simulink model "ADMIRE"  (R2021b)
settings: Solver=ode4  StartTime=0.0  StopTime=100  FixedStep=1e-2  RelTol=1e-3
undefined symbols (not defined in the file or in its folder): admireDB, Earth, WGS84
libraries: simulink_extras x112, simulink x27, aerolibutil x4, dspsigops x4, aerolibfltsims x3, sharedtransform x2, aerolibtransform2 x2, aerolibatmos2 x1, matrix_library x1, sharedutil x1, aerolibanimutils x1, vrlib x1
(part 5 of 15)

== system ADMIRE/Aircraft/Aerodynamics/NormalForceCoefficient/MachRegion3/Cncai ==
  in_bus : Inport
  Bus Selector : BusSelector  OutputSignals=AeroIn_Bus.angleOfAttack_deg,AeroIn_Bus.cai
  CNCAI_CAI_ALFA : Lookup_n-D  BreakpointsForDimension1=admireDB.aerodata_sym.CNCAI.breakpoints.ALFA  BreakpointsForDimension2=admireDB.aerodata_sym.CNCAI.breakpoints.CAI  BreakpointsForDimension3=[5, 7]  Table=admireDB.aerodata_sym.CNCAI.newTable  ExtrapMethod=Clip  InternalRulePriority=Speed  RndMeth=Simplest  InputSameDT=on
      settings: InputPortMap=u0,u1
  Cncai : Outport
  wires:
  CNCAI_CAI_ALFA/1 -> Cncai/1
  in_bus/1 -> Bus Selector/1  "in_bus"
  Bus Selector/2 -> CNCAI_CAI_ALFA/2  "<cai>"
  Bus Selector/1 -> CNCAI_CAI_ALFA/1  "<angleOfAttack_deg>"

== system ADMIRE/Aircraft/Aerodynamics/NormalForceCoefficient/MachRegion3/Cndedn ==
  Constant : Constant  Value=0
  Cndedn : Outport
  wires:
  Constant/1 -> Cndedn/1

== system ADMIRE/Aircraft/Aerodynamics/NormalForceCoefficient/MachRegion3/Cndei ==
  in_bus : Inport
  Bus Selector : BusSelector  OutputSignals=AeroIn_Bus.angleOfAttack_deg,AeroIn_Bus.dEI,AeroIn_Bus.mach_nd,eieff,AeroIn_Bus.qacorr
  CNEDEI_QA_M : Lookup_n-D  BreakpointsForDimension1=admireDB.aerodata_sym.CNEDEI.breakpoints.M  BreakpointsForDimension2=admireDB.aerodata_sym.CNEDEI.breakpoints.QA  BreakpointsForDimension3=[5, 7]  Table=admireDB.aerodata_sym.CNEDEI.newTable  ExtrapMethod=Clip  InternalRulePriority=Speed  RndMeth=Simplest  InputSameDT=on
      settings: InputPortMap=u0,u1
  Product : Product
  Subsystem : Subsystem
  Cndei : Outport
  wires:
  Product/1 -> Cndei/1
  Subsystem/1(Out1) -> Product/1
  Bus Selector/1 -> Subsystem/1(<angleOfAttack_deg>)  "<angleOfAttack_deg>"
  Bus Selector/2 -> Subsystem/2(<dEI>)  "<dEI>"
  Bus Selector/4 -> Subsystem/4(<eieff>)  "<eieff>"
  in_bus/1 -> Bus Selector/1  "in_bus"
  Bus Selector/5 -> CNEDEI_QA_M/2  "<qacorr>"
  Bus Selector/3 -> Subsystem/3(<mach_nd>), CNEDEI_QA_M/1  "<mach_nd>"
  CNEDEI_QA_M/1 -> Product/2

== system ADMIRE/Aircraft/Aerodynamics/NormalForceCoefficient/MachRegion3/Cndey ==
  in_bus : Inport
  Bus Selector : BusSelector  OutputSignals=AeroIn_Bus.angleOfAttack_deg,AeroIn_Bus.dEY,AeroIn_Bus.mach_nd,eieff,AeroIn_Bus.qacorr
  CNEDEY_QA_M : Lookup_n-D  BreakpointsForDimension1=admireDB.aerodata_sym.CNEDEY.breakpoints.M  BreakpointsForDimension2=admireDB.aerodata_sym.CNEDEY.breakpoints.QA  BreakpointsForDimension3=[5, 7]  Table=admireDB.aerodata_sym.CNEDEY.newTable  ExtrapMethod=Clip  InternalRulePriority=Speed  RndMeth=Simplest  InputSameDT=on
      settings: InputPortMap=u0,u1
  Product : Product
  Subsystem : Subsystem
  Cndey : Outport
  wires:
  CNEDEY_QA_M/1 -> Product/2
  Bus Selector/3 -> Subsystem/3(<mach_nd>), CNEDEY_QA_M/1  "<mach_nd>"
  Bus Selector/5 -> CNEDEY_QA_M/2  "<qacorr>"
  in_bus/1 -> Bus Selector/1  "in_bus"
  Bus Selector/4 -> Subsystem/4(<eieff>)  "<eieff>"
  Bus Selector/2 -> Subsystem/2(<dEI>)  "<dEY>"
  Bus Selector/1 -> Subsystem/1(<angleOfAttack_deg>)  "<angleOfAttack_deg>"
  Subsystem/1(Out1) -> Product/1
  Product/1 -> Cndey/1

== system ADMIRE/Aircraft/Aerodynamics/NormalForceCoefficient/MachRegion3/Cndle ==
  in_bus : Inport
  Bus Selector : BusSelector  OutputSignals=AeroIn_Bus.angleOfAttack_deg,AeroIn_Bus.mach_nd,AeroIn_Bus.lef_deg
  CNMDLEA_ALFA_DLE_M : Lookup_n-D  NumberOfTableDimensions=3  BreakpointsForDimension1=admireDB.aerodata_sym.CNMDLEA.breakpoints.ALFA  BreakpointsForDimension2=admireDB.aerodata_sym.CNMDLEA.breakpoints.DLE  BreakpointsForDimension3=admireDB.aerodata_sym.CNMDLEA.breakpoints.M  Table=admireDB.aerodata_sym.CNMDLEA.newTable  ExtrapMethod=Clip  InternalRulePriority=Speed  RndMeth=Simplest  InputSameDT=on
      settings: InputPortMap=u0,u1,u2
  Cndle : Outport
  wires:
  CNMDLEA_ALFA_DLE_M/1 -> Cndle/1
  Bus Selector/3 -> CNMDLEA_ALFA_DLE_M/3  "<lef_deg>"
  Bus Selector/2 -> CNMDLEA_ALFA_DLE_M/2  "<mach_nd>"
  Bus Selector/1 -> CNMDLEA_ALFA_DLE_M/1  "<angleOfAttack_deg>"
  in_bus/1 -> Bus Selector/1  "in_bus"

== system ADMIRE/Aircraft/Aerodynamics/NormalForceCoefficient/MachRegion3/Cndn ==
  in_bus : Inport
  Bus Selector : BusSelector  OutputSignals=AeroIn_Bus.dN,AeroIn_Bus.angleOfAttack_deg,AeroIn_Bus.mach_nd,AeroIn_Bus.qacorr
  CNDNH_M_DN_ALFA : Lookup_n-D  NumberOfTableDimensions=3  BreakpointsForDimension1=admireDB.aerodata_sym.CNDNH.breakpoints.M  BreakpointsForDimension2=admireDB.aerodata_sym.CNDNH.breakpoints.DN  BreakpointsForDimension3=admireDB.aerodata_sym.CNDNH.breakpoints.ALFA  Table=admireDB.aerodata_sym.CNDNH.newTable  ExtrapMethod=Clip  InternalRulePriority=Speed  RndMeth=Simplest  InputSameDT=on
      settings: InputPortMap=u0,u1,u2
  CNEDN_QA_M : Lookup_n-D  BreakpointsForDimension1=admireDB.aerodata_sym.CNEDN.breakpoints.M  BreakpointsForDimension2=admireDB.aerodata_sym.CNEDN.breakpoints.QA  BreakpointsForDimension3=[5, 7]  Table=admireDB.aerodata_sym.CNEDN.newTable  ExtrapMethod=Clip  InternalRulePriority=Speed  RndMeth=Simplest  InputSameDT=on
      settings: InputPortMap=u0,u1
  Product : Product
  Cndn : Outport
  wires:
  in_bus/1 -> Bus Selector/1  "in_bus"
  Bus Selector/1 -> CNDNH_M_DN_ALFA/2  "<dN>"
  Bus Selector/2 -> CNDNH_M_DN_ALFA/3  "<angleOfAttack_deg>"
  Bus Selector/4 -> CNEDN_QA_M/2  "<qacorr>"
  Bus Selector/3 -> CNDNH_M_DN_ALFA/1, CNEDN_QA_M/1  "<mach_nd>"
  CNEDN_QA_M/1 -> Product/2
  CNDNH_M_DN_ALFA/1 -> Product/1
  Product/1 -> Cndn/1

== system ADMIRE/Aircraft/Aerodynamics/NormalForceCoefficient/MachRegion3/Cnhigh ==
  Constant : Constant  Value=0
  Cnhigh : Outport
  wires:
  Constant/1 -> Cnhigh/1

== system ADMIRE/Aircraft/Aerodynamics/NormalForceCoefficient/MachRegion3/Cnlg ==
  in_bus : Inport
  Abs : Abs
  Bus Selector : BusSelector  OutputSignals=AeroIn_Bus.angleOfAttack_deg,AeroIn_Bus.angleOfSideslip_deg,AeroIn_Bus.lg_bool
  CNLST_BETA_ALFA : Lookup_n-D  BreakpointsForDimension1=admireDB.aerodata_sym.CNLST.breakpoints.ALFA  BreakpointsForDimension2=admireDB.aerodata_sym.CNLST.breakpoints.BETA  BreakpointsForDimension3=[5, 7]  Table=admireDB.aerodata_sym.CNLST.newTable  ExtrapMethod=Clip  InternalRulePriority=Speed  RndMeth=Simplest  InputSameDT=on
      settings: InputPortMap=u0,u1
  Product : Product
  Cnlg : Outport
  wires:
  Product/1 -> Cnlg/1
  in_bus/1 -> Bus Selector/1  "in_bus"
  Bus Selector/2 -> Abs/1  "<angleOfSideslip_deg>"
  Bus Selector/1 -> CNLST_BETA_ALFA/1  "<angleOfAttack_deg>"
  Abs/1 -> CNLST_BETA_ALFA/2
  CNLST_BETA_ALFA/1 -> Product/1
  Bus Selector/3 -> Product/2  "<lg_bool>"

== system ADMIRE/Aircraft/Aerodynamics/NormalForceCoefficient/MachRegion3/Cnnz ==
  in_bus : Inport
  Bus Selector : BusSelector  OutputSignals=AeroIn_Bus.nz_g,AeroIn_Bus.mach_nd,AeroIn_Bus.qacorr
  CNENZ_QA_M : Lookup_n-D  BreakpointsForDimension1=admireDB.aerodata_sym.CNENZ.breakpoints.M  BreakpointsForDimension2=admireDB.aerodata_sym.CNENZ.breakpoints.QA  BreakpointsForDimension3=[5, 7]  Table=admireDB.aerodata_sym.CNENZ.newTable  ExtrapMethod=Clip  InternalRulePriority=Speed  RndMeth=Simplest  InputSameDT=on
      settings: InputPortMap=u0,u1
  Constant : Constant
  Product : Product
  Sum : Sum  Inputs=-+|
  Cnnz : Outport
  wires:
  Bus Selector/2 -> CNENZ_QA_M/1  "<mach_nd>"
  Bus Selector/3 -> CNENZ_QA_M/2  "<qacorr>"
  Bus Selector/1 -> Sum/2  "<nz_g>"
  in_bus/1 -> Bus Selector/1  "in_bus"
  Product/1 -> Cnnz/1
  Constant/1 -> Sum/1
  Sum/1 -> Product/1
  CNENZ_QA_M/1 -> Product/2

== system ADMIRE/Aircraft/Aerodynamics/NormalForceCoefficient/MachRegion3/Cnq ==
  in_bus : Inport
  Bus Selector : BusSelector  OutputSignals=AeroIn_Bus.angleOfAttack_deg,AeroIn_Bus.qc,AeroIn_Bus.mach_nd,AeroIn_Bus.qacorr
  CNEQ_QA_M : Lookup_n-D  BreakpointsForDimension1=admireDB.aerodata_sym.CNEQ.breakpoints.M  BreakpointsForDimension2=admireDB.aerodata_sym.CNEQ.breakpoints.QA  BreakpointsForDimension3=[5, 7]  Table=admireDB.aerodata_sym.CNEQ.newTable  ExtrapMethod=Clip  InternalRulePriority=Speed  RndMeth=Simplest  InputSameDT=on
      settings: InputPortMap=u0,u1
  CNQAM_ALFA_M : Lookup_n-D  BreakpointsForDimension1=admireDB.aerodata_sym.CNQAM.breakpoints.M  BreakpointsForDimension2=admireDB.aerodata_sym.CNQAM.breakpoints.ALFA  BreakpointsForDimension3=[5, 7]  Table=admireDB.aerodata_sym.CNQAM.newTable  ExtrapMethod=Clip  InternalRulePriority=Speed  RndMeth=Simplest  InputSameDT=on
      settings: InputPortMap=u0,u1
  Product : Product  Inputs=3
  Cnq : Outport
  wires:
  CNQAM_ALFA_M/1 -> Product/1
  Product/1 -> Cnq/1
  in_bus/1 -> Bus Selector/1  "in_bus"
  Bus Selector/1 -> CNQAM_ALFA_M/2  "<angleOfAttack_deg>"
  Bus Selector/4 -> CNEQ_QA_M/2  "<qacorr>"
  Bus Selector/3 -> CNEQ_QA_M/1, CNQAM_ALFA_M/1  "<mach_nd>"
  CNEQ_QA_M/1 -> Product/3
  Bus Selector/2 -> Product/2  "<qc>"

== system ADMIRE/Aircraft/Aerodynamics/NormalForceCoefficient/MachRegion3/Cnqd ==
  in_bus : Inport
  Bus Selector : BusSelector  OutputSignals=AeroIn_Bus.qd,AeroIn_Bus.mach_nd,AeroIn_Bus.qacorr
  CNEQD_QA_M : Lookup_n-D  BreakpointsForDimension1=admireDB.aerodata_sym.CNEQD.breakpoints.M  BreakpointsForDimension2=admireDB.aerodata_sym.CNEQD.breakpoints.QA  BreakpointsForDimension3=[5, 7]  Table=admireDB.aerodata_sym.CNEQD.newTable  ExtrapMethod=Clip  InternalRulePriority=Speed  RndMeth=Simplest  InputSameDT=on
      settings: InputPortMap=u0,u1
  Product : Product
  Cnqd : Outport
  wires:
  CNEQD_QA_M/1 -> Product/2
  Product/1 -> Cnqd/1
  in_bus/1 -> Bus Selector/1  "in_bus"
  Bus Selector/1 -> Product/1  "<qd>"
  Bus Selector/3 -> CNEQD_QA_M/2  "<qacorr>"
  Bus Selector/2 -> CNEQD_QA_M/1  "<mach_nd>"

== system ADMIRE/Aircraft/Aerodynamics/NormalForceCoefficient/MachRegion3/eoeff ==
  AeroIn_Bus : Inport
  Abs : Abs
  Bus Selector : BusSelector  OutputSignals=mach_nd,angleOfAttack_deg
  CNDEYODE_ALFA_M : Lookup_n-D  BreakpointsForDimension1=admireDB.aerodata_sym.CNDEYODE.breakpoints.M  BreakpointsForDimension2=admireDB.aerodata_sym.CNDEYODE.breakpoints.ALFA  BreakpointsForDimension3=[5, 7]  Table=admireDB.aerodata_sym.CNDEYODE.newTable  ExtrapMethod=Clip  InternalRulePriority=Speed  RndMeth=Simplest  InputSameDT=on
      settings: InputPortMap=u0,u1
  Constant : Constant
  Sum : Sum  Inputs=-+|
  eoeff : Outport
  eieff : Outport  Port=2
  wires:
  AeroIn_Bus/1 -> Bus Selector/1
  Bus Selector/1 -> CNDEYODE_ALFA_M/1  "<mach_nd>"
  Constant/1 -> Sum/2
  CNDEYODE_ALFA_M/1 -> Sum/1, eoeff/1
  Sum/1 -> eieff/1
  Bus Selector/2 -> Abs/1  "<angleOfAttack_deg>"
  Abs/1 -> CNDEYODE_ALFA_M/2

== system ADMIRE/Aircraft/Aerodynamics/PitchMomentCoefficient/MachRegion1/Cpmalfa ==
  in_bus : Inport
  Bus Selector : BusSelector  OutputSignals=AeroIn_Bus.angleOfAttack_deg,AeroIn_Bus.mach_nd,AeroIn_Bus.qacorr
  CPMDEAL_DE_ALFA : Lookup_n-D  BreakpointsForDimension1=admireDB.aerodata_sym.CPMDEAL.breakpoints.ALFA  BreakpointsForDimension2=admireDB.aerodata_sym.CPMDEAL.breakpoints.DE  BreakpointsForDimension3=[5, 7]  Table=admireDB.aerodata_sym.CPMDEAL.newTable  ExtrapMethod=Clip  InternalRulePriority=Speed  RndMeth=Simplest  InputSameDT=on
      settings: InputPortMap=u0,u1
  CPMEA_QA_M : Lookup_n-D  BreakpointsForDimension1=admireDB.aerodata_sym.CPMEA.breakpoints.M  BreakpointsForDimension2=admireDB.aerodata_sym.CPMEA.breakpoints.QA  BreakpointsForDimension3=[5, 7]  Table=admireDB.aerodata_sym.CPMEA.newTable  ExtrapMethod=Clip  InternalRulePriority=Speed  RndMeth=Simplest  InputSameDT=on
      settings: InputPortMap=u0,u1
  Degrees to Radians : simulink_extras/Transformations/Degrees to Radians
  Product : Product
  Sum1 : Sum  Inputs=|++
  dE_cnst : Constant  Value=0.0
  Cpmalfa : Outport
  wires:
  Degrees to Radians/1 -> Product/1
  CPMEA_QA_M/1 -> Product/2
  Bus Selector/2 -> CPMEA_QA_M/1  "<mach_nd>"
  Bus Selector/3 -> CPMEA_QA_M/2  "<qacorr>"
  dE_cnst/1 -> CPMDEAL_DE_ALFA/2
  Bus Selector/1 -> Degrees to Radians/1, CPMDEAL_DE_ALFA/1  "<angleOfAttack_deg>"
  in_bus/1 -> Bus Selector/1  "in_bus"
  Sum1/1 -> Cpmalfa/1
  CPMDEAL_DE_ALFA/1 -> Sum1/1
  Product/1 -> Sum1/2

== system ADMIRE/Aircraft/Aerodynamics/PitchMomentCoefficient/MachRegion1/Cpmalfad ==
  in_bus : Inport
  Abs : Abs
  Bus Selector : BusSelector  OutputSignals=AeroIn_Bus.mach_nd,AeroIn_Bus.angleOfAttack_deg,AeroIn_Bus.alfad
  CPMADAM_ALFA_M : Lookup_n-D  BreakpointsForDimension1=admireDB.aerodata_sym.CPMADAM.breakpoints.M  BreakpointsForDimension2=admireDB.aerodata_sym.CPMADAM.breakpoints.ALFA  BreakpointsForDimension3=[5, 7]  Table=admireDB.aerodata_sym.CPMADAM.newTable  ExtrapMethod=Clip  InternalRulePriority=Speed  RndMeth=Simplest  InputSameDT=on
      settings: InputPortMap=u0,u1
  Product : Product
  Cpmalfad : Outport
  wires:
  Product/1 -> Cpmalfad/1
  Bus Selector/3 -> Product/2  "<alfad>"
  CPMADAM_ALFA_M/1 -> Product/1
  Abs/1 -> CPMADAM_ALFA_M/2
  Bus Selector/1 -> CPMADAM_ALFA_M/1  "<mach_nd>"
  Bus Selector/2 -> Abs/1  "<angleOfAttack_deg>"
  in_bus/1 -> Bus Selector/1  "in_bus"

== system ADMIRE/Aircraft/Aerodynamics/PitchMomentCoefficient/MachRegion1/Cpmbasic ==
  in_bus : Inport
  Bus Selector : BusSelector  OutputSignals=AeroIn_Bus.mach_nd,AeroIn_Bus.qacorr
  CPMEZERO_QA_M : Lookup_n-D  BreakpointsForDimension1=admireDB.aerodata_sym.CPMEZERO.breakpoints.M  BreakpointsForDimension2=admireDB.aerodata_sym.CPMEZERO.breakpoints.QA  BreakpointsForDimension3=[5, 7]  Table=admireDB.aerodata_sym.CPMEZERO.newTable  ExtrapMethod=Clip  InternalRulePriority=Speed  RndMeth=Simplest  InputSameDT=on
      settings: InputPortMap=u0,u1
  CPMZERO_M : Lookup_n-D  NumberOfTableDimensions=1  BreakpointsForDimension1=admireDB.aerodata_sym.CPMZERO.breakpoints.M  BreakpointsForDimension3=[5, 7]  Table=admireDB.aerodata_sym.CPMZERO.newTable  ExtrapMethod=Clip  InternalRulePriority=Speed  RndMeth=Simplest  InputSameDT=on
  Sum1 : Sum  Inputs=|++
  Cpmbasic : Outport
  wires:
  CPMEZERO_QA_M/1 -> Sum1/2
  CPMZERO_M/1 -> Sum1/1
  Bus Selector/2 -> CPMEZERO_QA_M/2  "<qacorr>"
  Bus Selector/1 -> CPMZERO_M/1, CPMEZERO_QA_M/1  "<mach_nd>"
  Sum1/1 -> Cpmbasic/1
  in_bus/1 -> Bus Selector/1  "in_bus"

== system ADMIRE/Aircraft/Aerodynamics/PitchMomentCoefficient/MachRegion1/Cpmbeta ==
  in_bus : Inport
  Abs : Abs
  Bus Selector : BusSelector  OutputSignals=AeroIn_Bus.angleOfAttack_deg,AeroIn_Bus.dN,AeroIn_Bus.angleOfSideslip_deg
  CPMBETA_ALFA_DN_BETA : Lookup_n-D  NumberOfTableDimensions=3  BreakpointsForDimension1=admireDB.aerodata_sym.CPMBETA.breakpoints.ALFA  BreakpointsForDimension2=admireDB.aerodata_sym.CPMBETA.breakpoints.DN  BreakpointsForDimension3=admireDB.aerodata_sym.CPMBETA.breakpoints.BETA  Table=admireDB.aerodata_sym.CPMBETA.newTable  ExtrapMethod=Clip  InternalRulePriority=Speed  RndMeth=Simplest  InputSameDT=on
      settings: InputPortMap=u0,u1,u2
  Cpmbeta : Outport
  wires:
  CPMBETA_ALFA_DN_BETA/1 -> Cpmbeta/1
  Abs/1 -> CPMBETA_ALFA_DN_BETA/3
  Bus Selector/3 -> Abs/1  "<angleOfSideslip_deg>"
  Bus Selector/1 -> CPMBETA_ALFA_DN_BETA/1  "<angleOfAttack_deg>"
  Bus Selector/2 -> CPMBETA_ALFA_DN_BETA/2  "<dN>"
  in_bus/1 -> Bus Selector/1  "in_bus"

== system ADMIRE/Aircraft/Aerodynamics/PitchMomentCoefficient/MachRegion1/Cpmcai ==
  in_bus : Inport
  Bus Selector : BusSelector  OutputSignals=AeroIn_Bus.angleOfAttack_deg,AeroIn_Bus.cai,AeroIn_Bus.dN
  CPMCAIDN_ALFA_CAI_DN : Lookup_n-D  NumberOfTableDimensions=3  BreakpointsForDimension1=admireDB.aerodata_sym.CPMCAIDN.breakpoints.ALFA  BreakpointsForDimension2=admireDB.aerodata_sym.CPMCAIDN.breakpoints.CAI  BreakpointsForDimension3=admireDB.aerodata_sym.CPMCAIDN.breakpoints.DN  Table=admireDB.aerodata_sym.CPMCAIDN.newTable  ExtrapMethod=Clip  InternalRulePriority=Speed  RndMeth=Simplest  InputSameDT=on
      settings: InputPortMap=u0,u1,u2
  CPMCAI_CAI_ALFA : Lookup_n-D  BreakpointsForDimension1=admireDB.aerodata_sym.CPMCAI.breakpoints.ALFA  BreakpointsForDimension2=admireDB.aerodata_sym.CPMCAI.breakpoints.CAI  BreakpointsForDimension3=[5, 7]  Table=admireDB.aerodata_sym.CPMCAI.newTable  ExtrapMethod=Clip  InternalRulePriority=Speed  RndMeth=Simplest  InputSameDT=on
      settings: InputPortMap=u0,u1
  Sum : Sum  Inputs=|++
  Cpmcai : Outport
  wires:
  CPMCAIDN_ALFA_CAI_DN/1 -> Sum/2
  Sum/1 -> Cpmcai/1
  in_bus/1 -> Bus Selector/1  "in_bus"
  Bus Selector/1 -> CPMCAI_CAI_ALFA/1, CPMCAIDN_ALFA_CAI_DN/1  "<angleOfAttack_deg>"
  Bus Selector/2 -> CPMCAIDN_ALFA_CAI_DN/2, CPMCAI_CAI_ALFA/2  "<cai>"
  CPMCAI_CAI_ALFA/1 -> Sum/1
  Bus Selector/3 -> CPMCAIDN_ALFA_CAI_DN/3  "<dN>"

== system ADMIRE/Aircraft/Aerodynamics/PitchMomentCoefficient/MachRegion1/Cpmda ==
  in_bus : Inport
  Abs : Abs
  Abs1 : Abs
  Bus Selector : BusSelector  OutputSignals=AeroIn_Bus.angleOfAttack_deg,AeroIn_Bus.dAI,eieff,AeroIn_Bus.dAY,eoeff
  CPMDAAL_DA_ALFA : Lookup_n-D  BreakpointsForDimension1=admireDB.aerodata_sym.CPMDAAL.breakpoints.ALFA  BreakpointsForDimension2=admireDB.aerodata_sym.CPMDAAL.breakpoints.DA  BreakpointsForDimension3=[5, 7]  Table=admireDB.aerodata_sym.CPMDAAL.newTable  ExtrapMethod=Clip  InternalRulePriority=Speed  RndMeth=Simplest  InputSameDT=on
      settings: InputPortMap=u0,u1
  CPMDAAL_DA_ALFA1 : Lookup_n-D  BreakpointsForDimension1=admireDB.aerodata_sym.CPMDAAL.breakpoints.ALFA  BreakpointsForDimension2=admireDB.aerodata_sym.CPMDAAL.breakpoints.DA  BreakpointsForDimension3=[5, 7]  Table=admireDB.aerodata_sym.CPMDAAL.newTable  ExtrapMethod=Clip  InternalRulePriority=Speed  RndMeth=Simplest  InputSameDT=on
      settings: InputPortMap=u0,u1
  Product : Product
  Product1 : Product
  Sum : Sum  Inputs=|++
  Cpmda : Outport
  wires:
  Abs1/1 -> CPMDAAL_DA_ALFA1/2
  Product1/1 -> Sum/2
  Product/1 -> Sum/1
  CPMDAAL_DA_ALFA1/1 -> Product1/1
  Bus Selector/3 -> Product/2  "<eieff>"
  CPMDAAL_DA_ALFA/1 -> Product/1
  Bus Selector/5 -> Product1/2  "<eoeff>"
  Bus Selector/4 -> Abs1/1  "<dAY>"
  Abs/1 -> CPMDAAL_DA_ALFA/2
  Bus Selector/2 -> Abs/1  "<dAI>"
  Bus Selector/1 -> CPMDAAL_DA_ALFA/1, CPMDAAL_DA_ALFA1/1  "<angleOfAttack_deg>"
  in_bus/1 -> Bus Selector/1  "in_bus"
  Sum/1 -> Cpmda/1

== system ADMIRE/Aircraft/Aerodynamics/PitchMomentCoefficient/MachRegion1/Cpmdedn ==
  in_bus : Inport
  Bus Selector : BusSelector  OutputSignals=AeroIn_Bus.angleOfAttack_deg,AeroIn_Bus.dE,AeroIn_Bus.dN
  CPMDNDE_ALFA_DE_DN : Lookup_n-D  NumberOfTableDimensions=3  BreakpointsForDimension1=admireDB.aerodata_sym.CPMDNDE.breakpoints.ALFA  BreakpointsForDimension2=admireDB.aerodata_sym.CPMDNDE.breakpoints.DE  BreakpointsForDimension3=admireDB.aerodata_sym.CPMDNDE.breakpoints.DN  Table=admireDB.aerodata_sym.CPMDNDE.newTable  ExtrapMethod=Clip  InternalRulePriority=Speed  RndMeth=Simplest  InputSameDT=on
      settings: InputPortMap=u0,u1,u2
  Cpmdedn : Outport
  wires:
  CPMDNDE_ALFA_DE_DN/1 -> Cpmdedn/1
  Bus Selector/3 -> CPMDNDE_ALFA_DE_DN/3  "<dN>"
  Bus Selector/2 -> CPMDNDE_ALFA_DE_DN/2  "<dE>"
  Bus Selector/1 -> CPMDNDE_ALFA_DE_DN/1  "<angleOfAttack_deg>"
  in_bus/1 -> Bus Selector/1  "in_bus"

== system ADMIRE/Aircraft/Aerodynamics/PitchMomentCoefficient/MachRegion1/Cpmdei ==
  in_bus : Inport
  Bus Selector : BusSelector  OutputSignals=AeroIn_Bus.dEI,AeroIn_Bus.angleOfAttack_deg,eieff,AeroIn_Bus.mach_nd,AeroIn_Bus.qacorr
  CPMEDEI_QA_M : Lookup_n-D  BreakpointsForDimension1=admireDB.aerodata_sym.CPMEDEI.breakpoints.M  BreakpointsForDimension2=admireDB.aerodata_sym.CPMEDEI.breakpoints.QA  BreakpointsForDimension3=[5, 7]  Table=admireDB.aerodata_sym.CPMEDEI.newTable  ExtrapMethod=Clip  InternalRulePriority=Speed  RndMeth=Simplest  InputSameDT=on
      settings: InputPortMap=u0,u1
  Product : Product
  Subsystem : Subsystem
  Cpmdei : Outport
  wires:
  Product/1 -> Cpmdei/1
  Subsystem/1(Out1) -> Product/1
  CPMEDEI_QA_M/1 -> Product/2
  Bus Selector/4 -> CPMEDEI_QA_M/1  "<mach_nd>"
  Bus Selector/3 -> Subsystem/3(<eieff>)  "<eieff>"
  Bus Selector/2 -> Subsystem/2(<angleOfAttack_deg>)  "<angleOfAttack_deg>"
  Bus Selector/1 -> Subsystem/1(<dEI>)  "<dEI>"
  Bus Selector/5 -> CPMEDEI_QA_M/2  "<qacorr>"
  in_bus/1 -> Bus Selector/1  "in_bus"

== system ADMIRE/Aircraft/Aerodynamics/PitchMomentCoefficient/MachRegion1/Cpmdey ==
  in_bus : Inport
  Bus Selector : BusSelector  OutputSignals=AeroIn_Bus.dEY,AeroIn_Bus.angleOfAttack_deg,eoeff,AeroIn_Bus.mach_nd,AeroIn_Bus.qacorr
  CPMEDEY_QA_M : Lookup_n-D  BreakpointsForDimension1=admireDB.aerodata_sym.CPMEDEY.breakpoints.M  BreakpointsForDimension2=admireDB.aerodata_sym.CPMEDEY.breakpoints.QA  BreakpointsForDimension3=[5, 7]  Table=admireDB.aerodata_sym.CPMEDEY.newTable  ExtrapMethod=Clip  InternalRulePriority=Speed  RndMeth=Simplest  InputSameDT=on
      settings: InputPortMap=u0,u1
  Product : Product
  Subsystem : Subsystem
  Cpmdey : Outport
  wires:
  in_bus/1 -> Bus Selector/1  "in_bus"
  Bus Selector/5 -> CPMEDEY_QA_M/2  "<qacorr>"
  Bus Selector/1 -> Subsystem/1(dEY)  "<dEY>"
  Bus Selector/2 -> Subsystem/2(angleOfAttack_deg)  "<angleOfAttack_deg>"
  Bus Selector/3 -> Subsystem/3(eoeff)  "<eoeff>"
  Bus Selector/4 -> CPMEDEY_QA_M/1  "<mach_nd>"
  CPMEDEY_QA_M/1 -> Product/2
  Subsystem/1(Out1) -> Product/1
  Product/1 -> Cpmdey/1

== system ADMIRE/Aircraft/Aerodynamics/PitchMomentCoefficient/MachRegion1/Cpmdle ==
  in_bus : Inport
  Bus Selector : BusSelector  OutputSignals=AeroIn_Bus.angleOfAttack_deg,AeroIn_Bus.dE,AeroIn_Bus.dN,AeroIn_Bus.lef_deg,AeroIn_Bus.qacorr,AeroIn_Bus.mach_nd
  Degrees to Radians : simulink_extras/Transformations/Degrees to Radians
  Product : Product
  Subsystem : Subsystem
  Subsystem1 : Subsystem
  Sum : Sum  Inputs=|++
  Cpmdle : Outport
  wires:
  Subsystem1/1(Out1) -> Product/1
  Bus Selector/6 -> Subsystem1/2(<mach_nd>)  "<mach_nd>"
  Bus Selector/5 -> Subsystem1/1(<qacorr>)  "<qacorr>"
  Sum/1 -> Cpmdle/1
  Subsystem/1(Out1) -> Sum/1
  Product/1 -> Sum/2
  Degrees to Radians/1 -> Product/2
  Bus Selector/4 -> Subsystem/4(<lef_deg>), Degrees to Radians/1  "<lef_deg>"
  Bus Selector/3 -> Subsystem/3(<dN>)  "<dN>"
  Bus Selector/2 -> Subsystem/2(<dE>)  "<dE>"
  Bus Selector/1 -> Subsystem/1(<angleOfAttack_deg>)  "<angleOfAttack_deg>"
  in_bus/1 -> Bus Selector/1  "in_bus"

== system ADMIRE/Aircraft/Aerodynamics/PitchMomentCoefficient/MachRegion1/Cpmdn ==
  in_bus : Inport
  Bus Selector : BusSelector  OutputSignals=AeroIn_Bus.angleOfAttack_deg,AeroIn_Bus.dN,AeroIn_Bus.mach_nd,AeroIn_Bus.qacorr
  CPMDNAL_DN_ALFA : Lookup_n-D  BreakpointsForDimension1=admireDB.aerodata_sym.CPMDNAL.breakpoints.ALFA  BreakpointsForDimension2=admireDB.aerodata_sym.CPMDNAL.breakpoints.DN  BreakpointsForDimension3=[5, 7]  Table=admireDB.aerodata_sym.CPMDNAL.newTable  ExtrapMethod=Clip  InternalRulePriority=Speed  RndMeth=Simplest  InputSameDT=on
      settings: InputPortMap=u0,u1
  CPMEDN_QA_M : Lookup_n-D  BreakpointsForDimension1=admireDB.aerodata_sym.CPMEDN.breakpoints.M  BreakpointsForDimension2=admireDB.aerodata_sym.CPMEDN.breakpoints.QA  BreakpointsForDimension3=[5, 7]  Table=admireDB.aerodata_sym.CPMEDN.newTable  ExtrapMethod=Clip  InternalRulePriority=Speed  RndMeth=Simplest  InputSameDT=on
      settings: InputPortMap=u0,u1
  Product : Product
  Cpmdn : Outport
  wires:
  CPMDNAL_DN_ALFA/1 -> Product/1
  CPMEDN_QA_M/1 -> Product/2
  Bus Selector/3 -> CPMEDN_QA_M/1  "<mach_nd>"
  Bus Selector/4 -> CPMEDN_QA_M/2  "<qacorr>"
  Bus Selector/2 -> CPMDNAL_DN_ALFA/2  "<dN>"
  Bus Selector/1 -> CPMDNAL_DN_ALFA/1  "<angleOfAttack_deg>"
  in_bus/1 -> Bus Selector/1  "in_bus"
  Product/1 -> Cpmdn/1

== system ADMIRE/Aircraft/Aerodynamics/PitchMomentCoefficient/MachRegion1/Cpmhigh ==
  in_bus : Inport
  Bus Selector : BusSelector  OutputSignals=AeroIn_Bus.angleOfAttack_deg,AeroIn_Bus.dN,AeroIn_Bus.dE
  CPMHDE_DE_ALFA : Lookup_n-D  BreakpointsForDimension1=admireDB.aerodata_high.CPMHDE.breakpoints.ALFA  BreakpointsForDimension2=admireDB.aerodata_high.CPMHDE.breakpoints.DE  BreakpointsForDimension3=[5, 7]  Table=admireDB.aerodata_high.CPMHDE.newTable  ExtrapMethod=Clip  InternalRulePriority=Speed  RndMeth=Simplest  InputSameDT=on
      settings: InputPortMap=u0,u1
  CPMHDN_DN_ALFA : Lookup_n-D  BreakpointsForDimension1=admireDB.aerodata_high.CPMHDN.breakpoints.ALFA  BreakpointsForDimension2=admireDB.aerodata_high.CPMHDN.breakpoints.DN  BreakpointsForDimension3=[5, 7]  Table=admireDB.aerodata_high.CPMHDN.newTable  ExtrapMethod=Clip  InternalRulePriority=Speed  RndMeth=Simplest  InputSameDT=on
      settings: InputPortMap=u0,u1
  CPMHZERO_ALFA : Lookup_n-D  NumberOfTableDimensions=1  BreakpointsForDimension1=admireDB.aerodata_high.CPMHZERO.breakpoints.ALFA  BreakpointsForDimension3=[5, 7]  Table=admireDB.aerodata_high.CPMHZERO.newTable  ExtrapMethod=Clip  InternalRulePriority=Speed  RndMeth=Simplest  InputSameDT=on
  Sum : Sum  Inputs=+++
  Cpmhigh : Outport
  wires:
  CPMHZERO_ALFA/1 -> Sum/1
  CPMHDE_DE_ALFA/1 -> Sum/3
  CPMHDN_DN_ALFA/1 -> Sum/2
  Bus Selector/3 -> CPMHDE_DE_ALFA/2  "<dE>"
  Bus Selector/2 -> CPMHDN_DN_ALFA/2  "<dN>"
  Bus Selector/1 -> CPMHZERO_ALFA/1, CPMHDN_DN_ALFA/1, CPMHDE_DE_ALFA/1  "<angleOfAttack_deg>"
  Sum/1 -> Cpmhigh/1
  in_bus/1 -> Bus Selector/1  "in_bus"

== system ADMIRE/Aircraft/Aerodynamics/PitchMomentCoefficient/MachRegion1/Cpmlg ==
  in_bus : Inport
  Abs : Abs
  Bus Selector : BusSelector  OutputSignals=AeroIn_Bus.angleOfAttack_deg,AeroIn_Bus.angleOfSideslip_deg,AeroIn_Bus.lg_bool
  CPMLST_BETA_ALFA : Lookup_n-D  BreakpointsForDimension1=admireDB.aerodata_sym.CPMLST.breakpoints.ALFA  BreakpointsForDimension2=admireDB.aerodata_sym.CPMLST.breakpoints.BETA  BreakpointsForDimension3=[5, 7]  Table=admireDB.aerodata_sym.CPMLST.newTable  ExtrapMethod=Clip  InternalRulePriority=Speed  RndMeth=Simplest  InputSameDT=on
      settings: InputPortMap=u0,u1
  Product : Product
  Cpmlg : Outport
  wires:
  Abs/1 -> CPMLST_BETA_ALFA/2
  Bus Selector/3 -> Product/2  "<lg_bool>"
  CPMLST_BETA_ALFA/1 -> Product/1
  Bus Selector/2 -> Abs/1  "<angleOfSideslip_deg>"
  Bus Selector/1 -> CPMLST_BETA_ALFA/1  "<angleOfAttack_deg>"
  in_bus/1 -> Bus Selector/1  "in_bus"
  Product/1 -> Cpmlg/1

== system ADMIRE/Aircraft/Aerodynamics/PitchMomentCoefficient/MachRegion1/Cpmnz ==
  in_bus : Inport
  Bus Selector : BusSelector  OutputSignals=AeroIn_Bus.nz_g,AeroIn_Bus.mach_nd,AeroIn_Bus.qacorr
  CPMENZ_QA_M : Lookup_n-D  BreakpointsForDimension1=admireDB.aerodata_sym.CPMENZ.breakpoints.M  BreakpointsForDimension2=admireDB.aerodata_sym.CPMENZ.breakpoints.QA  BreakpointsForDimension3=[5, 7]  Table=admireDB.aerodata_sym.CPMENZ.newTable  ExtrapMethod=Clip  InternalRulePriority=Speed  RndMeth=Simplest  InputSameDT=on
      settings: InputPortMap=u0,u1
  Constant : Constant
  Product : Product
  Sum : Sum  Inputs=-+|
  Cpmnz : Outport
  wires:
  CPMENZ_QA_M/1 -> Product/2
  Constant/1 -> Sum/1
  Bus Selector/1 -> Sum/2  "<nz_g>"
  Bus Selector/2 -> CPMENZ_QA_M/1  "<mach_nd>"
  Bus Selector/3 -> CPMENZ_QA_M/2  "<qacorr>"
  Product/1 -> Cpmnz/1
  Sum/1 -> Product/1
  in_bus/1 -> Bus Selector/1  "in_bus"

== system ADMIRE/Aircraft/Aerodynamics/PitchMomentCoefficient/MachRegion1/Cpmq ==
  in_bus : Inport
  Bus Selector : BusSelector  OutputSignals=AeroIn_Bus.angleOfAttack_deg,AeroIn_Bus.dN,AeroIn_Bus.mach_nd,AeroIn_Bus.qacorr,AeroIn_Bus.qc
  CPMEQ_QA_M : Lookup_n-D  BreakpointsForDimension1=admireDB.aerodata_sym.CPMEQ.breakpoints.M  BreakpointsForDimension2=admireDB.aerodata_sym.CPMEQ.breakpoints.QA  BreakpointsForDimension3=[5, 7]  Table=admireDB.aerodata_sym.CPMEQ.newTable  ExtrapMethod=Clip  InternalRulePriority=Speed  RndMeth=Simplest  InputSameDT=on
      settings: InputPortMap=u0,u1
  CPMQAL_ALFA : Lookup_n-D  NumberOfTableDimensions=1  BreakpointsForDimension1=admireDB.aerodata_sym.CPMQAL.breakpoints.ALFA  BreakpointsForDimension3=[5, 7]  Table=admireDB.aerodata_sym.CPMQAL.newTable  ExtrapMethod=Clip  InternalRulePriority=Speed  RndMeth=Simplest  InputSameDT=on
  CPMQDNAL_DN_ALFA : Lookup_n-D  BreakpointsForDimension1=admireDB.aerodata_sym.CPMQDNAL.breakpoints.ALFA  BreakpointsForDimension2=admireDB.aerodata_sym.CPMQDNAL.breakpoints.DN  BreakpointsForDimension3=[5, 7]  Table=admireDB.aerodata_sym.CPMQDNAL.newTable  ExtrapMethod=Clip  InternalRulePriority=Speed  RndMeth=Simplest  InputSameDT=on
      settings: InputPortMap=u0,u1
  Product : Product  Inputs=3
  Sum : Sum  Inputs=++|
  Cpmq : Outport
  wires:
  Bus Selector/5 -> Product/3  "<qc>"
  CPMEQ_QA_M/1 -> Product/2
  Bus Selector/3 -> CPMEQ_QA_M/1  "<mach_nd>"
  Bus Selector/4 -> CPMEQ_QA_M/2  "<qacorr>"
  CPMQAL_ALFA/1 -> Sum/1
  CPMQDNAL_DN_ALFA/1 -> Sum/2
  Bus Selector/2 -> CPMQDNAL_DN_ALFA/2  "<dN>"
  Bus Selector/1 -> CPMQAL_ALFA/1, CPMQDNAL_DN_ALFA/1  "<angleOfAttack_deg>"
  in_bus/1 -> Bus Selector/1  "in_bus"
  Sum/1 -> Product/1
  Product/1 -> Cpmq/1

== system ADMIRE/Aircraft/Aerodynamics/PitchMomentCoefficient/MachRegion1/Cpmqd ==
  in_bus : Inport
  Bus Selector : BusSelector  OutputSignals=AeroIn_Bus.qd,AeroIn_Bus.mach_nd,AeroIn_Bus.qacorr
  CPMEQD_QA_M : Lookup_n-D  BreakpointsForDimension1=admireDB.aerodata_sym.CPMEQD.breakpoints.M  BreakpointsForDimension2=admireDB.aerodata_sym.CPMEQD.breakpoints.QA  BreakpointsForDimension3=[5, 7]  Table=admireDB.aerodata_sym.CPMEQD.newTable  ExtrapMethod=Clip  InternalRulePriority=Speed  RndMeth=Simplest  InputSameDT=on
      settings: InputPortMap=u0,u1
  Product : Product
  Cpmqd : Outport
  wires:
  in_bus/1 -> Bus Selector/1  "in_bus"
  Product/1 -> Cpmqd/1
  Bus Selector/3 -> CPMEQD_QA_M/2  "<qacorr>"
  Bus Selector/2 -> CPMEQD_QA_M/1  "<mach_nd>"
  Bus Selector/1 -> Product/1  "<qd>"
  CPMEQD_QA_M/1 -> Product/2

== system ADMIRE/Aircraft/Aerodynamics/PitchMomentCoefficient/MachRegion1/eoeff ==
  AeroIn_Bus : Inport
  Abs : Abs
  Bus Selector : BusSelector  OutputSignals=mach_nd,angleOfAttack_deg
  CPMDEYOD_ALFA_M : Lookup_n-D  BreakpointsForDimension1=admireDB.aerodata_sym.CPMDEYOD.breakpoints.M  BreakpointsForDimension2=admireDB.aerodata_sym.CPMDEYOD.breakpoints.ALFA  BreakpointsForDimension3=[5, 7]  Table=admireDB.aerodata_sym.CPMDEYOD.newTable  ExtrapMethod=Clip  InternalRulePriority=Speed  RndMeth=Simplest  InputSameDT=on
      settings: InputPortMap=u0,u1
  Constant : Constant
  Sum : Sum  Inputs=-+|
  eoeff : Outport
  eieff : Outport  Port=2
  wires:
  Abs/1 -> CPMDEYOD_ALFA_M/2
  Bus Selector/2 -> Abs/1  "<angleOfAttack_deg>"
  Sum/1 -> eieff/1
  CPMDEYOD_ALFA_M/1 -> eoeff/1, Sum/1
  Constant/1 -> Sum/2
  Bus Selector/1 -> CPMDEYOD_ALFA_M/1  "<mach_nd>"
  AeroIn_Bus/1 -> Bus Selector/1

== system ADMIRE/Aircraft/Aerodynamics/PitchMomentCoefficient/MachRegion2/Cpmalfa ==
  in_bus : Inport
  Bus Selector : BusSelector  OutputSignals=AeroIn_Bus.angleOfAttack_deg,AeroIn_Bus.tflow,AeroIn_Bus.tfhigh,AeroIn_Bus.mach_nd,AeroIn_Bus.qacorr
  CPMDEAL : Subsystem
  CPMEA_QA_M : Lookup_n-D  BreakpointsForDimension1=admireDB.aerodata_sym.CPMEA.breakpoints.M  BreakpointsForDimension2=admireDB.aerodata_sym.CPMEA.breakpoints.QA  BreakpointsForDimension3=[5, 7]  Table=admireDB.aerodata_sym.CPMEA.newTable  ExtrapMethod=Clip  InternalRulePriority=Speed  RndMeth=Simplest  InputSameDT=on
      settings: InputPortMap=u0,u1
  CPMMDEA : Subsystem
  Degrees to Radians : simulink_extras/Transformations/Degrees to Radians
  Product : Product
  Sum1 : Sum  Inputs=+++
  Cpmalfa : Outport
  wires:
  Degrees to Radians/1 -> Product/2
  CPMMDEA/1(Out1) -> Sum1/2
  Bus Selector/3 -> CPMMDEA/1(tfhigh)  "<tfhigh>"
  CPMDEAL/1(Out1) -> Sum1/1
  Bus Selector/2 -> CPMDEAL/2(tflow)  "<tflow>"
  Product/1 -> Sum1/3
  Sum1/1 -> Cpmalfa/1
  in_bus/1 -> Bus Selector/1  "in_bus"
  Bus Selector/1 -> CPMMDEA/2(angleOfAttack_deg), Degrees to Radians/1, CPMDEAL/1(angleOfAttack_deg)  "<angleOfAttack_deg>"
  Bus Selector/4 -> CPMEA_QA_M/1  "<mach_nd>"
  Bus Selector/5 -> CPMEA_QA_M/2  "<qacorr>"
  CPMEA_QA_M/1 -> Product/1

== system ADMIRE/Aircraft/Aerodynamics/PitchMomentCoefficient/MachRegion2/Cpmalfad ==
  in_bus : Inport
  Abs : Abs
  Bus Selector : BusSelector  OutputSignals=AeroIn_Bus.mach_nd,AeroIn_Bus.angleOfAttack_deg,AeroIn_Bus.alfad
  CPMADAM_ALFA_M : Lookup_n-D  BreakpointsForDimension1=admireDB.aerodata_sym.CPMADAM.breakpoints.M  BreakpointsForDimension2=admireDB.aerodata_sym.CPMADAM.breakpoints.ALFA  BreakpointsForDimension3=[5, 7]  Table=admireDB.aerodata_sym.CPMADAM.newTable  ExtrapMethod=Clip  InternalRulePriority=Speed  RndMeth=Simplest  InputSameDT=on
      settings: InputPortMap=u0,u1
  Product : Product
  Cpmalfad : Outport
  wires:
  in_bus/1 -> Bus Selector/1  "in_bus"
  Bus Selector/2 -> Abs/1  "<angleOfAttack_deg>"
  Bus Selector/1 -> CPMADAM_ALFA_M/1  "<mach_nd>"
  Abs/1 -> CPMADAM_ALFA_M/2
  CPMADAM_ALFA_M/1 -> Product/1
  Bus Selector/3 -> Product/2  "<alfad>"
  Product/1 -> Cpmalfad/1

== system ADMIRE/Aircraft/Aerodynamics/PitchMomentCoefficient/MachRegion2/Cpmbasic ==
  in_bus : Inport
  Bus Selector : BusSelector  OutputSignals=AeroIn_Bus.mach_nd,AeroIn_Bus.qacorr
  CPMEZERO_QA_M : Lookup_n-D  BreakpointsForDimension1=admireDB.aerodata_sym.CPMEZERO.breakpoints.M  BreakpointsForDimension2=admireDB.aerodata_sym.CPMEZERO.breakpoints.QA  BreakpointsForDimension3=[5, 7]  Table=admireDB.aerodata_sym.CPMEZERO.newTable  ExtrapMethod=Clip  InternalRulePriority=Speed  RndMeth=Simplest  InputSameDT=on
      settings: InputPortMap=u0,u1
  CPMZERO_M : Lookup_n-D  NumberOfTableDimensions=1  BreakpointsForDimension1=admireDB.aerodata_sym.CPMZERO.breakpoints.M  BreakpointsForDimension3=[5, 7]  Table=admireDB.aerodata_sym.CPMZERO.newTable  ExtrapMethod=Clip  InternalRulePriority=Speed  RndMeth=Simplest  InputSameDT=on
  Sum1 : Sum  Inputs=|++
  Cpmbasic : Outport
  wires:
  in_bus/1 -> Bus Selector/1  "in_bus"
  Sum1/1 -> Cpmbasic/1
  Bus Selector/1 -> CPMZERO_M/1, CPMEZERO_QA_M/1  "<mach_nd>"
  Bus Selector/2 -> CPMEZERO_QA_M/2  "<qacorr>"
  CPMZERO_M/1 -> Sum1/1
  CPMEZERO_QA_M/1 -> Sum1/2

== system ADMIRE/Aircraft/Aerodynamics/PitchMomentCoefficient/MachRegion2/Cpmbeta ==
  in_bus : Inport
  Abs : Abs
  Bus Selector : BusSelector  OutputSignals=AeroIn_Bus.tflow,AeroIn_Bus.angleOfAttack_deg,AeroIn_Bus.dN,AeroIn_Bus.angleOfSideslip_deg
  CPMBETA_ALFA_DN_BETA : Lookup_n-D  NumberOfTableDimensions=3  BreakpointsForDimension1=admireDB.aerodata_sym.CPMBETA.breakpoints.ALFA  BreakpointsForDimension2=admireDB.aerodata_sym.CPMBETA.breakpoints.DN  BreakpointsForDimension3=admireDB.aerodata_sym.CPMBETA.breakpoints.BETA  Table=admireDB.aerodata_sym.CPMBETA.newTable  ExtrapMethod=Clip  InternalRulePriority=Speed  RndMeth=Simplest  InputSameDT=on
      settings: InputPortMap=u0,u1,u2
  Product : Product
  Cpmbeta : Outport
  wires:
  Bus Selector/1 -> Product/1  "<tflow>"
  Product/1 -> Cpmbeta/1
  in_bus/1 -> Bus Selector/1  "in_bus"
  Bus Selector/3 -> CPMBETA_ALFA_DN_BETA/2  "<dN>"
  Bus Selector/2 -> CPMBETA_ALFA_DN_BETA/1  "<angleOfAttack_deg>"
  Bus Selector/4 -> Abs/1  "<angleOfSideslip_deg>"
  Abs/1 -> CPMBETA_ALFA_DN_BETA/3
  CPMBETA_ALFA_DN_BETA/1 -> Product/2

== system ADMIRE/Aircraft/Aerodynamics/PitchMomentCoefficient/MachRegion2/Cpmcai ==
  in_bus : Inport
  Bus Selector : BusSelector  OutputSignals=AeroIn_Bus.angleOfAttack_deg,AeroIn_Bus.cai,AeroIn_Bus.dN
  CPMCAIDN_ALFA_CAI_DN : Lookup_n-D  NumberOfTableDimensions=3  BreakpointsForDimension1=admireDB.aerodata_sym.CPMCAIDN.breakpoints.ALFA  BreakpointsForDimension2=admireDB.aerodata_sym.CPMCAIDN.breakpoints.CAI  BreakpointsForDimension3=admireDB.aerodata_sym.CPMCAIDN.breakpoints.DN  Table=admireDB.aerodata_sym.CPMCAIDN.newTable  ExtrapMethod=Clip  InternalRulePriority=Speed  RndMeth=Simplest  InputSameDT=on
      settings: InputPortMap=u0,u1,u2
  CPMCAI_CAI_ALFA : Lookup_n-D  BreakpointsForDimension1=admireDB.aerodata_sym.CPMCAI.breakpoints.ALFA  BreakpointsForDimension2=admireDB.aerodata_sym.CPMCAI.breakpoints.CAI  BreakpointsForDimension3=[5, 7]  Table=admireDB.aerodata_sym.CPMCAI.newTable  ExtrapMethod=Clip  InternalRulePriority=Speed  RndMeth=Simplest  InputSameDT=on
      settings: InputPortMap=u0,u1
  Sum : Sum  Inputs=|++
  Cpmcai : Outport
  wires:
  Bus Selector/3 -> CPMCAIDN_ALFA_CAI_DN/3  "<dN>"
  CPMCAI_CAI_ALFA/1 -> Sum/1
  Bus Selector/2 -> CPMCAIDN_ALFA_CAI_DN/2, CPMCAI_CAI_ALFA/2  "<cai>"
  Bus Selector/1 -> CPMCAI_CAI_ALFA/1, CPMCAIDN_ALFA_CAI_DN/1  "<angleOfAttack_deg>"
  in_bus/1 -> Bus Selector/1  "in_bus"
  Sum/1 -> Cpmcai/1
  CPMCAIDN_ALFA_CAI_DN/1 -> Sum/2

== system ADMIRE/Aircraft/Aerodynamics/PitchMomentCoefficient/MachRegion2/Cpmda ==
  in_bus : Inport
  Bus Selector : BusSelector  OutputSignals=AeroIn_Bus.tflow,AeroIn_Bus.dAI,AeroIn_Bus.angleOfAttack_deg,eiefflow,AeroIn_Bus.dAY,eoefflow
  CPMDAAL : Subsystem
  Product : Product
  Cpmda : Outport
  wires:
  Product/1 -> Cpmda/1
  CPMDAAL/1(Out1) -> Product/2
  Bus Selector/6 -> CPMDAAL/5(eoefflow)  "<eoefflow>"
  Bus Selector/5 -> CPMDAAL/4(dAY)  "<dAY>"
  Bus Selector/4 -> CPMDAAL/3(eiefflow)  "<eiefflow>"
  Bus Selector/3 -> CPMDAAL/2(angleOfAttack_deg)  "<angleOfAttack_deg>"
  Bus Selector/2 -> CPMDAAL/1(dAI)  "<dAI>"
  Bus Selector/1 -> Product/1  "<tflow>"
  in_bus/1 -> Bus Selector/1  "in_bus"

== system ADMIRE/Aircraft/Aerodynamics/PitchMomentCoefficient/MachRegion2/Cpmdedn ==
  in_bus : Inport
  Bus Selector : BusSelector  OutputSignals=AeroIn_Bus.angleOfAttack_deg,AeroIn_Bus.dE,AeroIn_Bus.dN,AeroIn_Bus.tflow
  CPMDNDE_ALFA_DE_DN : Lookup_n-D  NumberOfTableDimensions=3  BreakpointsForDimension1=admireDB.aerodata_sym.CPMDNDE.breakpoints.ALFA  BreakpointsForDimension2=admireDB.aerodata_sym.CPMDNDE.breakpoints.DE  BreakpointsForDimension3=admireDB.aerodata_sym.CPMDNDE.breakpoints.DN  Table=admireDB.aerodata_sym.CPMDNDE.newTable  ExtrapMethod=Clip  InternalRulePriority=Speed  RndMeth=Simplest  InputSameDT=on
      settings: InputPortMap=u0,u1,u2
  Product : Product
  Cpmdedn : Outport
  wires:
  Product/1 -> Cpmdedn/1
  Bus Selector/4 -> Product/2  "<tflow>"
  in_bus/1 -> Bus Selector/1  "in_bus"
  Bus Selector/1 -> CPMDNDE_ALFA_DE_DN/1  "<angleOfAttack_deg>"
  Bus Selector/2 -> CPMDNDE_ALFA_DE_DN/2  "<dE>"
  Bus Selector/3 -> CPMDNDE_ALFA_DE_DN/3  "<dN>"
  CPMDNDE_ALFA_DE_DN/1 -> Product/1

== system ADMIRE/Aircraft/Aerodynamics/PitchMomentCoefficient/MachRegion2/Cpmdei ==
  in_bus : Inport
  Bus Selector : BusSelector  OutputSignals=eieff,AeroIn_Bus.dEI,AeroIn_Bus.angleOfAttack_deg,AeroIn_Bus.tflow,AeroIn_Bus.tfhigh,AeroIn_Bus.mach_nd,AeroIn_Bus.qacorr
  CPMDEAL : Subsystem
  CPMEDEI_QA_M : Lookup_n-D  BreakpointsForDimension1=admireDB.aerodata_sym.CPMEDEI.breakpoints.M  BreakpointsForDimension2=admireDB.aerodata_sym.CPMEDEI.breakpoints.QA  BreakpointsForDimension3=[5, 7]  Table=admireDB.aerodata_sym.CPMEDEI.newTable  ExtrapMethod=Clip  InternalRulePriority=Speed  RndMeth=Simplest  InputSameDT=on
      settings: InputPortMap=u0,u1
  CPMMDEA : Subsystem
  Product : Product  Inputs=3
  Sum : Sum  Inputs=|++
  Cpmdei : Outport
  wires:
  Product/1 -> Cpmdei/1
  [P2] -> Product/3
  [P1] -> Product/1
  Sum/1 -> Product/2
  CPMEDEI_QA_M/1 -> [P2]
  CPMDEAL/1(Out1) -> Sum/1
  CPMMDEA/1(Out1) -> Sum/2
  Bus Selector/5 -> CPMMDEA/1(tfhigh)  "<tfhigh>"
  Bus Selector/4 -> CPMDEAL/3(tflow)  "<tflow>"
  in_bus/1 -> Bus Selector/1  "in_bus"
  Bus Selector/7 -> CPMEDEI_QA_M/2  "<qacorr>"
  Bus Selector/2 -> CPMMDEA/3(dEI), CPMDEAL/1(dEI)  "<dEI>"
  Bus Selector/3 -> CPMDEAL/2(angleOfAttack_deg), CPMMDEA/2(angleOfAttack_deg)  "<angleOfAttack_deg>"
  Bus Selector/1 -> [P1]  "<eieff>"
  Bus Selector/6 -> CPMEDEI_QA_M/1  "<mach_nd>"

== system ADMIRE/Aircraft/Aerodynamics/PitchMomentCoefficient/MachRegion2/Cpmdey ==
  in_bus : Inport
  Bus Selector : BusSelector  OutputSignals=eoeff,AeroIn_Bus.dEY,AeroIn_Bus.angleOfAttack_deg,AeroIn_Bus.tflow,AeroIn_Bus.tfhigh,AeroIn_Bus.mach_nd,AeroIn_Bus.qacorr
  CPMDEAL : Subsystem
  CPMEDEY_QA_M : Lookup_n-D  BreakpointsForDimension1=admireDB.aerodata_sym.CPMEDEY.breakpoints.M  BreakpointsForDimension2=admireDB.aerodata_sym.CPMEDEY.breakpoints.QA  BreakpointsForDimension3=[5, 7]  Table=admireDB.aerodata_sym.CPMEDEY.newTable  ExtrapMethod=Clip  InternalRulePriority=Speed  RndMeth=Simplest  InputSameDT=on
      settings: InputPortMap=u0,u1
  CPMMDEA : Subsystem
  Product : Product  Inputs=3
  Sum : Sum  Inputs=|++
  Cpmdey : Outport
  wires:
  Bus Selector/6 -> CPMEDEY_QA_M/1  "<mach_nd>"
  Bus Selector/1 -> [P1]  "<eoeff>"
  Bus Selector/3 -> CPMMDEA/2(angleOfAttack_deg), CPMDEAL/2(angleOfAttack_deg)  "<angleOfAttack_deg>"
  Bus Selector/2 -> CPMDEAL/1(dEI), CPMMDEA/3(dEI)  "<dEY>"
  Bus Selector/7 -> CPMEDEY_QA_M/2  "<qacorr>"
  in_bus/1 -> Bus Selector/1  "in_bus"
  Bus Selector/4 -> CPMDEAL/3(tflow)  "<tflow>"
  Bus Selector/5 -> CPMMDEA/1(tfhigh)  "<tfhigh>"
  CPMMDEA/1(Out1) -> Sum/2
  CPMDEAL/1(Out1) -> Sum/1
  CPMEDEY_QA_M/1 -> [P2]
  Sum/1 -> Product/2
  [P1] -> Product/1
  [P2] -> Product/3
  Product/1 -> Cpmdey/1

== system ADMIRE/Aircraft/Aerodynamics/PitchMomentCoefficient/MachRegion2/Cpmdle ==
  in_bus : Inport
  Bus Selector : BusSelector  OutputSignals=AeroIn_Bus.angleOfAttack_deg,AeroIn_Bus.dE,AeroIn_Bus.dN,AeroIn_Bus.tflow,AeroIn_Bus.tfhigh,AeroIn_Bus.lef_deg,AeroIn_Bus.qacorr,AeroIn_Bus.mach_nd
  Degrees to Radians : simulink_extras/Transformations/Degrees to Radians
  Product : Product
  Subsystem : Subsystem
  Subsystem1 : Subsystem
  Sum : Sum  Inputs=|++
  Cpmdle : Outport
  wires:
  Bus Selector/5 -> Subsystem/5(tfhigh)  "<tfhigh>"
  Bus Selector/4 -> Subsystem/4(tflow)  "<tflow>"
  in_bus/1 -> Bus Selector/1  "in_bus"
  Bus Selector/1 -> Subsystem/1(angleOfAttack_deg)  "<angleOfAttack_deg>"
  Bus Selector/2 -> Subsystem/2(dE)  "<dE>"
  Bus Selector/3 -> Subsystem/3(dN)  "<dN>"
  Bus Selector/6 -> Degrees to Radians/1, Subsystem/6(lef_deg)  "<lef_deg>"
  Degrees to Radians/1 -> Product/2
  Product/1 -> Sum/2
  Subsystem/1(Out1) -> Sum/1
  Sum/1 -> Cpmdle/1
  Bus Selector/7 -> Subsystem1/1(qacorr)  "<qacorr>"
  Bus Selector/8 -> Subsystem1/2(mach_nd)  "<mach_nd>"
  Subsystem1/1(Out1) -> Product/1

== system ADMIRE/Aircraft/Aerodynamics/PitchMomentCoefficient/MachRegion2/Cpmdn ==
  in_bus : Inport
  Bus Selector : BusSelector  OutputSignals=AeroIn_Bus.dN,AeroIn_Bus.angleOfAttack_deg,AeroIn_Bus.tflow,AeroIn_Bus.tfhigh,AeroIn_Bus.mach_nd,AeroIn_Bus.qacorr
  CPMDNAL_CPMMDNA : Subsystem
  CPMEDN_QA_M : Lookup_n-D  BreakpointsForDimension1=admireDB.aerodata_sym.CPMEDN.breakpoints.M  BreakpointsForDimension2=admireDB.aerodata_sym.CPMEDN.breakpoints.QA  BreakpointsForDimension3=[5, 7]  Table=admireDB.aerodata_sym.CPMEDN.newTable  ExtrapMethod=Clip  InternalRulePriority=Speed  RndMeth=Simplest  InputSameDT=on
      settings: InputPortMap=u0,u1
  Product : Product
  Cpmdn : Outport
  wires:
  CPMDNAL_CPMMDNA/1(Out1) -> Product/1
  Bus Selector/2 -> CPMDNAL_CPMMDNA/2(angleOfAttack_deg)  "<angleOfAttack_deg>"
  Bus Selector/1 -> CPMDNAL_CPMMDNA/1(dN)  "<dN>"
  Bus Selector/4 -> CPMDNAL_CPMMDNA/4(tfhigh)  "<tfhigh>"
  Bus Selector/3 -> CPMDNAL_CPMMDNA/3(tflow)  "<tflow>"
  Product/1 -> Cpmdn/1
  in_bus/1 -> Bus Selector/1  "in_bus"
  Bus Selector/6 -> CPMEDN_QA_M/2  "<qacorr>"
  Bus Selector/5 -> CPMEDN_QA_M/1  "<mach_nd>"
  CPMEDN_QA_M/1 -> Product/2

== system ADMIRE/Aircraft/Aerodynamics/PitchMomentCoefficient/MachRegion2/Cpmhigh ==
  Constant : Constant  Value=0
  Cpmhigh : Outport
  wires:
  Constant/1 -> Cpmhigh/1

== system ADMIRE/Aircraft/Aerodynamics/PitchMomentCoefficient/MachRegion2/Cpmlg ==
  in_bus : Inport
  Abs : Abs
  Bus Selector : BusSelector  OutputSignals=AeroIn_Bus.angleOfAttack_deg,AeroIn_Bus.angleOfSideslip_deg,AeroIn_Bus.lg_bool
  CPMLST_BETA_ALFA : Lookup_n-D  BreakpointsForDimension1=admireDB.aerodata_sym.CPMLST.breakpoints.ALFA  BreakpointsForDimension2=admireDB.aerodata_sym.CPMLST.breakpoints.BETA  BreakpointsForDimension3=[5, 7]  Table=admireDB.aerodata_sym.CPMLST.newTable  ExtrapMethod=Clip  InternalRulePriority=Speed  RndMeth=Simplest  InputSameDT=on
      settings: InputPortMap=u0,u1
  Product : Product
  Cpmlg : Outport
  wires:
  Product/1 -> Cpmlg/1
  in_bus/1 -> Bus Selector/1  "in_bus"
  Bus Selector/1 -> CPMLST_BETA_ALFA/1  "<angleOfAttack_deg>"
  Bus Selector/2 -> Abs/1  "<angleOfSideslip_deg>"
  CPMLST_BETA_ALFA/1 -> Product/1
  Bus Selector/3 -> Product/2  "<lg_bool>"
  Abs/1 -> CPMLST_BETA_ALFA/2

== system ADMIRE/Aircraft/Aerodynamics/PitchMomentCoefficient/MachRegion2/Cpmnz ==
  in_bus : Inport
  Bus Selector : BusSelector  OutputSignals=AeroIn_Bus.nz_g,AeroIn_Bus.mach_nd,AeroIn_Bus.qacorr
  CPMENZ_QA_M : Lookup_n-D  BreakpointsForDimension1=admireDB.aerodata_sym.CPMENZ.breakpoints.M  BreakpointsForDimension2=admireDB.aerodata_sym.CPMENZ.breakpoints.QA  BreakpointsForDimension3=[5, 7]  Table=admireDB.aerodata_sym.CPMENZ.newTable  ExtrapMethod=Clip  InternalRulePriority=Speed  RndMeth=Simplest  InputSameDT=on
      settings: InputPortMap=u0,u1
  Constant : Constant
  Product : Product
  Sum : Sum  Inputs=-+|
  Cpmnz : Outport
  wires:
  in_bus/1 -> Bus Selector/1  "in_bus"
  Sum/1 -> Product/1
  Product/1 -> Cpmnz/1
  Bus Selector/3 -> CPMENZ_QA_M/2  "<qacorr>"
  Bus Selector/2 -> CPMENZ_QA_M/1  "<mach_nd>"
  Bus Selector/1 -> Sum/2  "<nz_g>"
  Constant/1 -> Sum/1
  CPMENZ_QA_M/1 -> Product/2

== system ADMIRE/Aircraft/Aerodynamics/PitchMomentCoefficient/MachRegion2/Cpmq ==
  in_bus : Inport
  Bus Selector : BusSelector  OutputSignals=AeroIn_Bus.tflow,AeroIn_Bus.angleOfAttack_deg,AeroIn_Bus.dN,AeroIn_Bus.tfhigh,AeroIn_Bus.mach_nd,AeroIn_Bus.qacorr,AeroIn_Bus.qc
  CPMEQ_QA_M : Lookup_n-D  BreakpointsForDimension1=admireDB.aerodata_sym.CPMEQ.breakpoints.M  BreakpointsForDimension2=admireDB.aerodata_sym.CPMEQ.breakpoints.QA  BreakpointsForDimension3=[5, 7]  Table=admireDB.aerodata_sym.CPMEQ.newTable  ExtrapMethod=Clip  InternalRulePriority=Speed  RndMeth=Simplest  InputSameDT=on
      settings: InputPortMap=u0,u1
  Product : Product  Inputs=3
  Subsystem : Subsystem
  Cpmq : Outport
  wires:
  Subsystem/1(Out1) -> Product/1
  Bus Selector/4 -> Subsystem/4(tfhigh)  "<tfhigh>"
  Bus Selector/3 -> Subsystem/3(dN)  "<dN>"
  Bus Selector/2 -> Subsystem/2(angleOfAttack_deg)  "<angleOfAttack_deg>"
  Bus Selector/1 -> Subsystem/1(tflow)  "<tflow>"
  Product/1 -> Cpmq/1
  in_bus/1 -> Bus Selector/1  "in_bus"
  Bus Selector/6 -> CPMEQ_QA_M/2  "<qacorr>"
  Bus Selector/5 -> CPMEQ_QA_M/1  "<mach_nd>"
  CPMEQ_QA_M/1 -> Product/2
  Bus Selector/7 -> Product/3  "<qc>"

== system ADMIRE/Aircraft/Aerodynamics/PitchMomentCoefficient/MachRegion2/Cpmqd ==
  in_bus : Inport
  Bus Selector : BusSelector  OutputSignals=AeroIn_Bus.qd,AeroIn_Bus.mach_nd,AeroIn_Bus.qacorr
  CPMEQD_QA_M : Lookup_n-D  BreakpointsForDimension1=admireDB.aerodata_sym.CPMEQD.breakpoints.M  BreakpointsForDimension2=admireDB.aerodata_sym.CPMEQD.breakpoints.QA  BreakpointsForDimension3=[5, 7]  Table=admireDB.aerodata_sym.CPMEQD.newTable  ExtrapMethod=Clip  InternalRulePriority=Speed  RndMeth=Simplest  InputSameDT=on
      settings: InputPortMap=u0,u1
  Product : Product
  Cpmqd : Outport
  wires:
  CPMEQD_QA_M/1 -> Product/2
  Bus Selector/1 -> Product/1  "<qd>"
  Bus Selector/2 -> CPMEQD_QA_M/1  "<mach_nd>"
  Bus Selector/3 -> CPMEQD_QA_M/2  "<qacorr>"
  Product/1 -> Cpmqd/1
  in_bus/1 -> Bus Selector/1  "in_bus"

== system ADMIRE/Aircraft/Aerodynamics/PitchMomentCoefficient/MachRegion2/eoeff ==
  AeroIn_Bus : Inport
  Abs : Abs
  Bus Selector : BusSelector  OutputSignals=mach_nd,angleOfAttack_deg
  CPMDEYOD_ALFA_M : Lookup_n-D  BreakpointsForDimension1=admireDB.aerodata_sym.CPMDEYOD.breakpoints.M  BreakpointsForDimension2=admireDB.aerodata_sym.CPMDEYOD.breakpoints.ALFA  BreakpointsForDimension3=[5, 7]  Table=admireDB.aerodata_sym.CPMDEYOD.newTable  ExtrapMethod=Clip  InternalRulePriority=Speed  RndMeth=Simplest  InputSameDT=on
      settings: InputPortMap=u0,u1
  CPMDEYOD_ALFA_M1 : Lookup_n-D  BreakpointsForDimension1=admireDB.aerodata_sym.CPMDEYOD.breakpoints.M  BreakpointsForDimension2=admireDB.aerodata_sym.CPMDEYOD.breakpoints.ALFA  BreakpointsForDimension3=[5, 7]  Table=admireDB.aerodata_sym.CPMDEYOD.newTable  ExtrapMethod=Clip  InternalRulePriority=Speed  RndMeth=Simplest  InputSameDT=on
      settings: InputPortMap=u0,u1
  Constant : Constant
  Constant1 : Constant  Value=0.4
  Constant2 : Constant
  Sum : Sum  Inputs=-+|
  Sum1 : Sum  Inputs=-+|
  eoeff : Outport
  eieff : Outport  Port=2
  eoefflow : Outport  Port=3
  eiefflow : Outport  Port=4
  wires:
  Constant1/1 -> CPMDEYOD_ALFA_M1/1
  Sum1/1 -> eiefflow/1
  CPMDEYOD_ALFA_M1/1 -> eoefflow/1, Sum1/1
  Constant2/1 -> Sum1/2
  Bus Selector/1 -> CPMDEYOD_ALFA_M/1  "<mach_nd>"
  AeroIn_Bus/1 -> Bus Selector/1
  Constant/1 -> Sum/2
  CPMDEYOD_ALFA_M/1 -> Sum/1, eoeff/1
  Sum/1 -> eieff/1
  Bus Selector/2 -> Abs/1  "<angleOfAttack_deg>"
  Abs/1 -> CPMDEYOD_ALFA_M/2, CPMDEYOD_ALFA_M1/2
